simulink model "model4"  (R2015a)
settings: Solver=ode4  StartTime=0.0  StopTime=t  FixedStep=T_s  RelTol=1e-3
values from neighbouring files (symbols this model uses):
  a = 9    [initm4.m]
  b = 27    [initm4.m]
  c = 27    [initm4.m]
  kbar = 100    [initm4.m]
  kx0 = 100    [initm4.m]
  kz0 = 100    [initm4.m]
  n = 100    [initm4.m]
  U = 0.2    [initm4.m]
settings Model: CovModelRefEnable=off  Creator=Subodh  LastModifiedBy=Subodh
settings DataIOCC: SaveFormat=Dataset
settings HardwareCC: ProdBitPerPointer=64  ProdLargestAtomicFloat=Float  ProdIntDivRoundTo=Zero  ProdEndianess=LittleEndian  ProdHWDeviceType=Specified

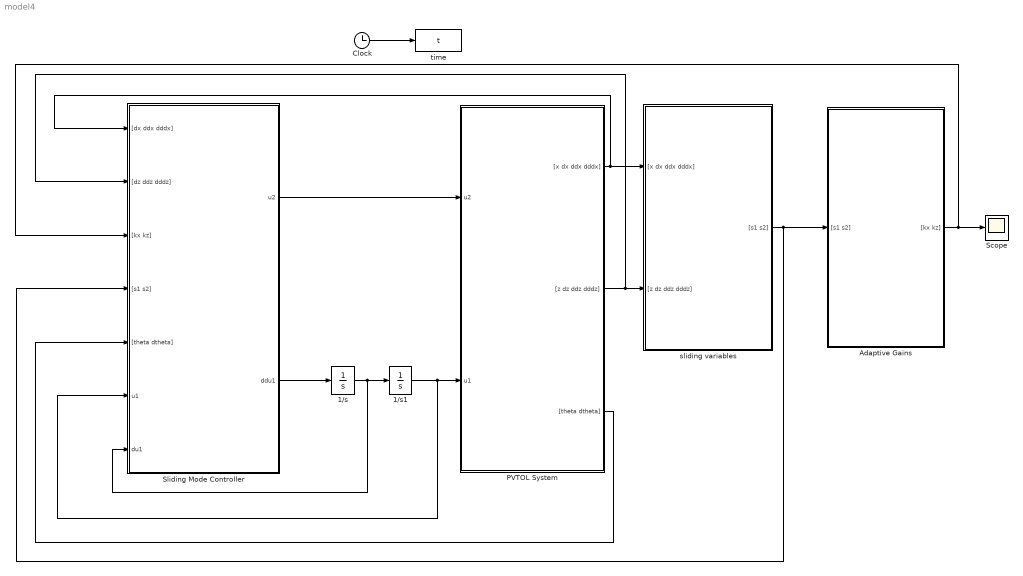
== system model4 ==
  1/s : Integrator
  1/s1 : Integrator  InitialCondition=0.1
  Adaptive Gains : Subsystem
  Clock : Clock
  PVTOL System : Subsystem
  Scope : Scope
      settings: TimeRange=auto  MaxDataPoints=5000  SaveToWorkspace=off  SaveName=ScopeData  YMin=249.24719  YMax=250.58278  SampleTime=-1
  Sliding Mode Controller : Subsystem
  sliding variables : Subsystem
  time : ToWorkspace  VariableName=t  SampleTime=-1
  wires:
  Clock/1 -> time/1
  PVTOL System/1("[x dx ddx dddx]") -> sliding variables/1("[x dx ddx dddx]"), Sliding Mode Controller/1("[dx ddx dddx]")
  PVTOL System/2("[z dz ddz dddz]") -> sliding variables/2("[z dz ddz dddz]"), Sliding Mode Controller/2("[dz ddz dddz]")
  1/s/1 -> Sliding Mode Controller/7(du1), 1/s1/1
  1/s1/1 -> Sliding Mode Controller/6(u1), PVTOL System/2(u1)
  Sliding Mode Controller/1(u2) -> PVTOL System/1(u2)
  Sliding Mode Controller/2(ddu1) -> 1/s/1
  sliding variables/1("[s1 s2]") -> Sliding Mode Controller/4("[s1 s2]"), Adaptive Gains/1("[s1 s2]")
  PVTOL System/3("[theta dtheta]") -> Sliding Mode Controller/5("[theta dtheta]")
  Adaptive Gains/1("[kx kz]") -> Scope/1, Sliding Mode Controller/3("[kx kz]")

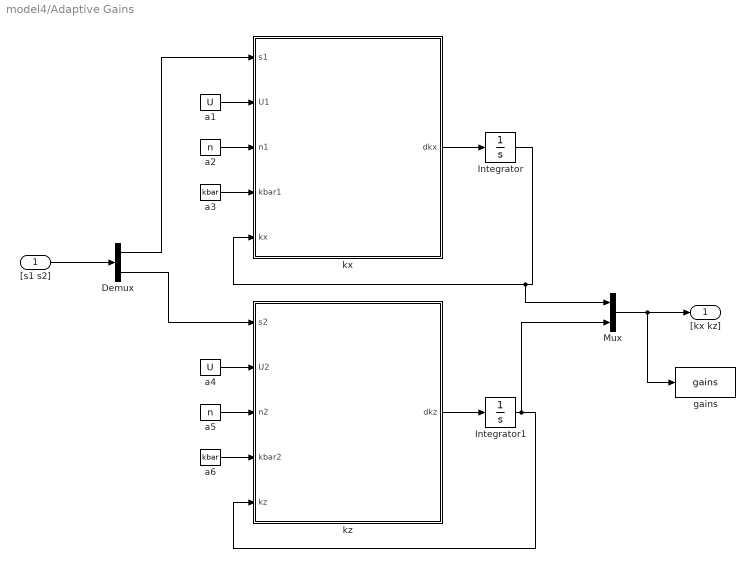
== system model4/Adaptive Gains ==
  "[s1 s2]" : Inport
  Demux : Demux  Outputs=2
  Integrator : Integrator  InitialCondition=kx0
  Integrator1 : Integrator  InitialCondition=kz0
  Mux : Mux  Inputs=2
  a1 : Constant  Value=U
  a2 : Constant  Value=n
  a3 : Constant  Value=kbar
  a4 : Constant  Value=U
  a5 : Constant  Value=n
  a6 : Constant  Value=kbar
  gains : ToWorkspace  VariableName=gains  SampleTime=-1
  kx : MATLAB Function  TreatAsAtomicUnit=on
      settings: PermitHierarchicalResolution=ParametersOnly
  kz : MATLAB Function  TreatAsAtomicUnit=on
      settings: PermitHierarchicalResolution=ParametersOnly
  "[kx kz]" : Outport
  wires:
  "[s1 s2]"/1 -> Demux/1
  Mux/1 -> gains/1, "[kx kz]"/1
  a2/1 -> kx/3(n1)
  a1/1 -> kx/2(U1)
  kx/1(dkx) -> Integrator/1
  a4/1 -> kz/2(U2)
  Demux/1 -> kx/1(s1)
  a5/1 -> kz/3(n2)
  a6/1 -> kz/4(kbar2)
  a3/1 -> kx/4(kbar1)
  kz/1(dkz) -> Integrator1/1
  Integrator/1 -> Mux/1, kx/5(kx)
  Integrator1/1 -> Mux/2, kz/5(kz)
  Demux/2 -> kz/1(s2)

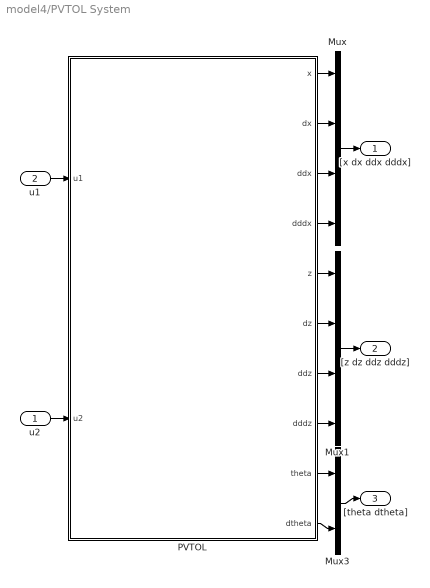
== system model4/PVTOL System ==
  u2 : Inport
  u1 : Inport  Port=2
  Mux : Mux
  Mux1 : Mux
  Mux3 : Mux  Inputs=2
  PVTOL : Subsystem
  "[x dx ddx dddx]" : Outport
  "[z dz ddz dddz]" : Outport  Port=2
  "[theta dtheta]" : Outport  Port=3
  wires:
  PVTOL/5(z) -> Mux1/1
  PVTOL/7(ddz) -> Mux1/3
  PVTOL/6(dz) -> Mux1/2
  PVTOL/2(dx) -> Mux/2
  u1/1 -> PVTOL/1(u1)
  Mux/1 -> "[x dx ddx dddx]"/1
  Mux3/1 -> "[theta dtheta]"/1
  u2/1 -> PVTOL/2(u2)
  Mux1/1 -> "[z dz ddz dddz]"/1
  PVTOL/3(ddx) -> Mux/3
  PVTOL/4(dddx) -> Mux/4
  PVTOL/8(dddz) -> Mux1/4
  PVTOL/1(x) -> Mux/1
  PVTOL/10(dtheta) -> Mux3/2
  PVTOL/9(theta) -> Mux3/1

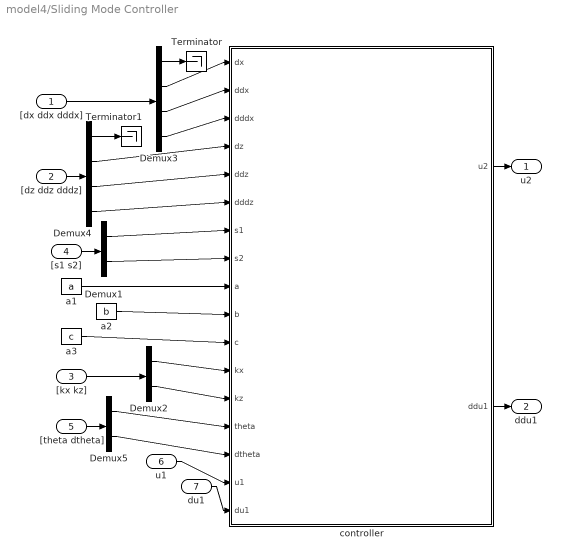
== system model4/Sliding Mode Controller ==
  "[dx ddx dddx]" : Inport
  "[dz ddz dddz]" : Inport  Port=2
  "[kx kz]" : Inport  Port=3
  "[s1 s2]" : Inport  Port=4
  "[theta dtheta]" : Inport  Port=5
  u1 : Inport  Port=6
  du1 : Inport  Port=7
  Demux1 : Demux  Outputs=2
  Demux2 : Demux  Outputs=2
  Demux3 : Demux
  Demux4 : Demux
  Demux5 : Demux  Outputs=2
  Terminator : Terminator
  Terminator1 : Terminator
  a1 : Constant  Value=a
  a2 : Constant  Value=b
  a3 : Constant  Value=c
  controller : MATLAB Function  TreatAsAtomicUnit=on
      settings: PermitHierarchicalResolution=ParametersOnly
  u2 : Outport
  ddu1 : Outport  Port=2
  wires:
  Demux4/2 -> controller/4(dz)
  Demux1/1 -> controller/7(s1)
  "[theta dtheta]"/1 -> Demux5/1
  Demux3/2 -> controller/1(dx)
  Demux5/2 -> controller/15(dtheta)
  "[dz ddz dddz]"/1 -> Demux4/1
  u1/1 -> controller/16(u1)
  controller/1(u2) -> u2/1
  du1/1 -> controller/17(du1)
  controller/2(ddu1) -> ddu1/1
  "[s1 s2]"/1 -> Demux1/1
  "[dx ddx dddx]"/1 -> Demux3/1
  Demux4/4 -> controller/6(dddz)
  Demux3/3 -> controller/2(ddx)
  Demux4/3 -> controller/5(ddz)
  Demux5/1 -> controller/14(theta)
  Demux3/1 -> Terminator/1
  Demux4/1 -> Terminator1/1
  Demux3/4 -> controller/3(dddx)
  a1/1 -> controller/9(a)
  a2/1 -> controller/10(b)
  a3/1 -> controller/11(c)
  Demux1/2 -> controller/8(s2)
  Demux2/1 -> controller/12(kx)
  Demux2/2 -> controller/13(kz)
  "[kx kz]"/1 -> Demux2/1

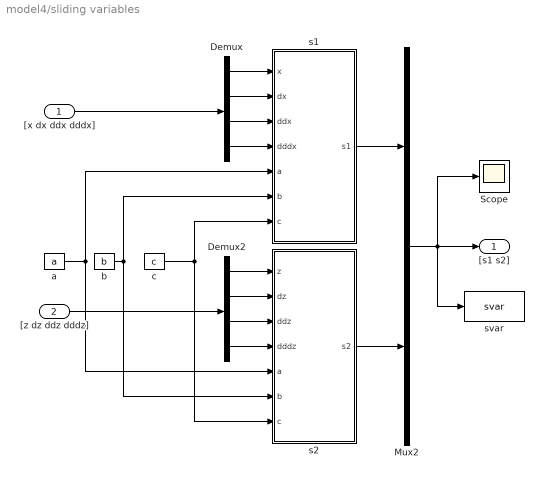
== system model4/sliding variables ==
  "[x dx ddx dddx]" : Inport
  "[z dz ddz dddz]" : Inport  Port=2
  Demux : Demux
  Demux2 : Demux
  Mux2 : Mux  Inputs=2
  Scope : Scope
      settings: TimeRange=auto  MaxDataPoints=5000  SaveToWorkspace=off  YMin=-7.16262  YMax=60.79585  SampleTime=-1
  a : Constant  Value=a
  b : Constant  Value=b
  c : Constant  Value=c
  s1 : MATLAB Function  TreatAsAtomicUnit=on
      settings: PermitHierarchicalResolution=ParametersOnly
  s2 : MATLAB Function  TreatAsAtomicUnit=on
      settings: PermitHierarchicalResolution=ParametersOnly
  svar : ToWorkspace  VariableName=svar  SampleTime=-1
  "[s1 s2]" : Outport
  wires:
  c/1 -> s1/7(c), s2/7(c)
  Demux/1 -> s1/1(x)
  s2/1(s2) -> Mux2/2
  Mux2/1 -> svar/1, Scope/1, "[s1 s2]"/1
  a/1 -> s2/5(a), s1/5(a)
  "[x dx ddx dddx]"/1 -> Demux/1
  "[z dz ddz dddz]"/1 -> Demux2/1
  Demux/4 -> s1/4(dddx)
  Demux/2 -> s1/2(dx)
  Demux/3 -> s1/3(ddx)
  Demux2/3 -> s2/3(ddz)
  Demux2/4 -> s2/4(dddz)
  Demux2/2 -> s2/2(dz)
  Demux2/1 -> s2/1(z)
  s1/1(s1) -> Mux2/1
  b/1 -> s2/6(b), s1/6(b)

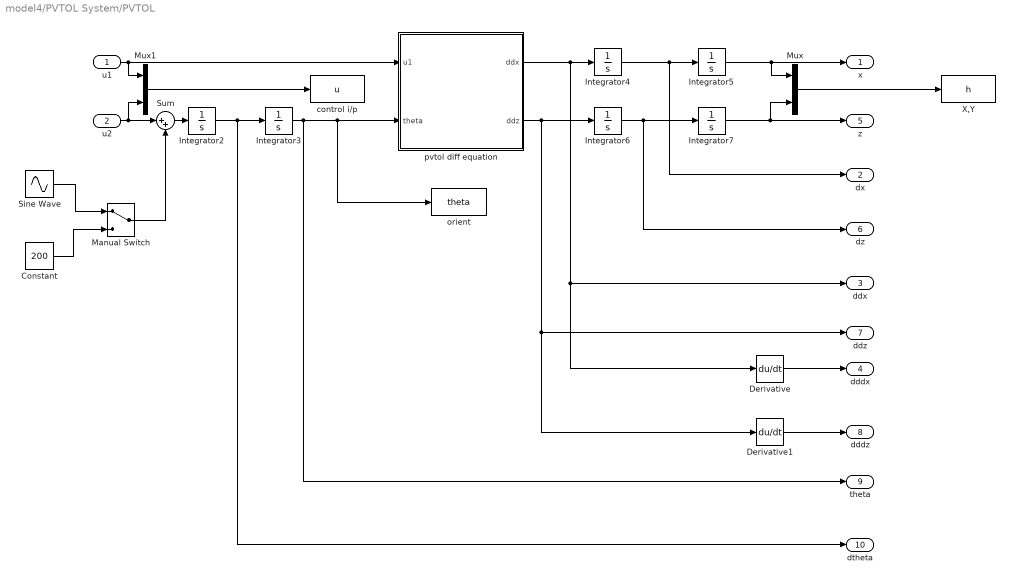
== system model4/PVTOL System/PVTOL ==
  u1 : Inport
  u2 : Inport  Port=2
  Constant : Constant  Value=200
  Derivative : Derivative
  Derivative1 : Derivative
  Integrator{2..4,6} (4 alike) : Integrator
  Integrator5 : Integrator  InitialCondition=1
  Integrator7 : Integrator  InitialCondition=2
  Manual Switch : ManualSwitch
  Mux : Mux  Inputs=2
  Mux1 : Mux  Inputs=2
  Sine Wave : Sin  Amplitude=200  SampleTime=0
  Sum : Sum  Inputs=|++
  X,Y : ToWorkspace  VariableName=h  SampleTime=-1
  control i/p : ToWorkspace  VariableName=u  SampleTime=-1
  orient : ToWorkspace  VariableName=theta  SampleTime=-1
  pvtol diff equation : MATLAB Function  TreatAsAtomicUnit=on
      settings: PermitHierarchicalResolution=ParametersOnly
  x : Outport
  dx : Outport  Port=2
  ddx : Outport  Port=3
  dddx : Outport  Port=4
  z : Outport  Port=5
  dz : Outport  Port=6
  ddz : Outport  Port=7
  dddz : Outport  Port=8
  theta : Outport  Port=9
  dtheta : Outport  Port=10
  wires:
  Integrator5/1 -> Mux/1, x/1
  pvtol diff equation/1(ddx) -> Derivative/1, ddx/1, Integrator4/1
  Integrator6/1 -> dz/1, Integrator7/1
  u1/1 -> Mux1/1, pvtol diff equation/1(u1)
  Integrator2/1 -> dtheta/1, Integrator3/1
  pvtol diff equation/2(ddz) -> Derivative1/1, ddz/1, Integrator6/1
  Integrator7/1 -> z/1, Mux/2
  Integrator4/1 -> dx/1, Integrator5/1
  Integrator3/1 -> orient/1, pvtol diff equation/2(theta), theta/1
  Sum/1 -> Integrator2/1
  Constant/1 -> Manual Switch/2
  Sine Wave/1 -> Manual Switch/1
  Derivative/1 -> dddx/1
  Derivative1/1 -> dddz/1
  Mux/1 -> X,Y/1
  Mux1/1 -> control i/p/1
  u2/1 -> Mux1/2, Sum/1
  Manual Switch/1 -> Sum/2

== matlab function model4/sliding variables/s1 ==
  data: x input; dx input; ddx input; s1 output; dddx input; a input; b input; c input
function s1= slidingVar1(x,dx,ddx,dddx,a,b,c)
%#codegen
s1=dddx+a*ddx+b*dx+c*x;
end

== matlab function model4/PVTOL System/PVTOL/pvtol diff equation ==
  data: u1 input; ddx output; theta input; ddz output
function [ddx,ddz] = system(u1,theta)
%#codegen
ddx=-u1*sin(theta);
ddz=u1*cos(theta)-1;
end

== matlab function model4/sliding variables/s2 ==
  data: z input; dz input; ddz input; s2 output; dddz input; a input; b input; c input
function s2= slidingVar2(z,dz,ddz,dddz,a,b,c)
%#codegen
s2=dddz+a*ddz+b*dz+c*z;
end

== matlab function model4/Sliding Mode Controller/controller ==
  data: u2 output; dx input; ddx input; ddu1 output; dddx input; dz input; ddz input; dddz input; s1 input; s2 input; a input; b input; c input; kx input; kz input; theta input; dtheta input; u1 input; du1 input
function [u2,ddu1]= Controller(dx,ddx,dddx,dz,ddz,dddz,s1,s2,a,b,c,kx,kz,theta,dtheta, u1,du1)
%#codegen
alpha=a*[dddx;dddz]+b*[ddx;ddz]+c*[dx;dz]+[u1*(dtheta^2)*sin(theta)-2*du1*dtheta*cos(theta);-u1*(dtheta^2)*cos(theta)-2*du1*dtheta*sin(theta)];
beta=[-sin(theta) -u1*cos(theta);cos(theta) -u1*sin(theta)];
u=inv(beta)*([-kx*sign(s1);-kz*sign(s2)]-alpha);
ddu1=u(1);
u2=u(2);
end

== matlab function model4/Adaptive Gains/kx ==
  data: s1 input; U1 input; n1 input; kbar1 input; kx input; dkx output
function dkx= gainX(s1,U1,n1,kbar1,kx)
%#codegen
if kx>n1
    dkx=kbar1*abs(s1)*sign(abs(s1)-U1);
else
    dkx=n1;
end
end

== matlab function model4/Adaptive Gains/kz ==
  data: s2 input; U2 input; n2 input; kbar2 input; kz input; dkz output
function dkz= gainZ(s2,U2,n2,kbar2,kz)
%#codegen
if kz>n2
    dkz=kbar2*abs(s2)*sign(abs(s2)-U2);
else
    dkz=n2;
end

end
